simulink model "kapitsa"  (R2023b)
settings: Solver=VariableStepAuto  StartTime=0.0  StopTime=10.0  MaxStep=1e-4  RelTol=1e-3
undefined symbols (not defined in the file): f, I, l, m
settings Model: Creator=B03-304  LastModifiedBy=B03-304

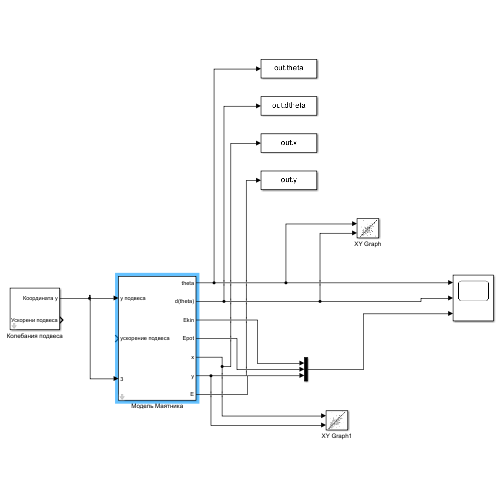
[thumbnail: Simulink's stored preview of the top-level diagram]
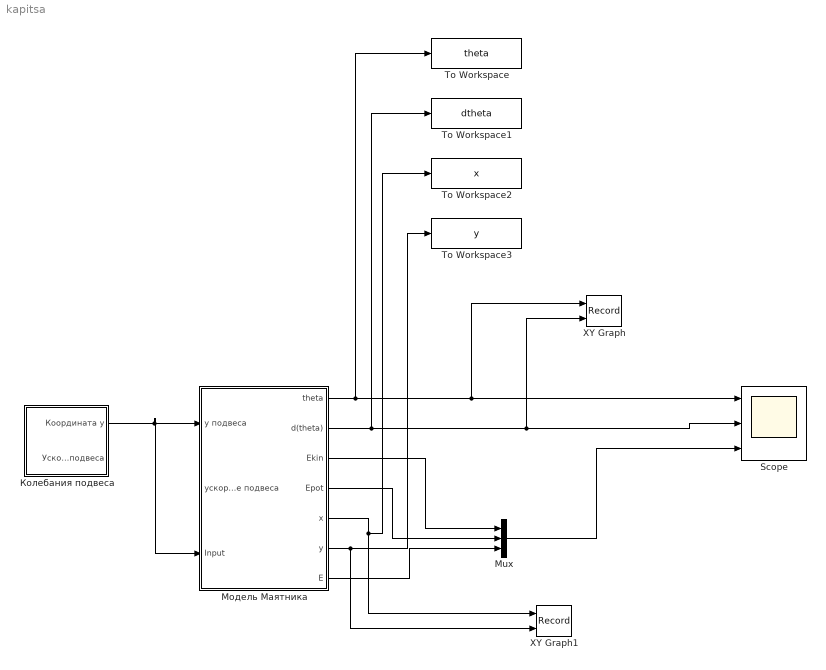
== system kapitsa ==
  Mux : Mux  Inputs=3
  Scope : Scope  NumInputPorts=3
  To Workspace : ToWorkspace  VariableName=theta  SampleTime=-1
  To Workspace1 : ToWorkspace  VariableName=dtheta  SampleTime=-1
  To Workspace2 : ToWorkspace  VariableName=x  SampleTime=-1
  To Workspace3 : ToWorkspace  VariableName=y  SampleTime=-1
  XY Graph : Record  FileSettingsInternal="{\"entries\":[{\"content\":{\"excelSettings\":{\"content\":{},\"type\":\"Streamout.ExcelSettings\"}},\"type\":\"Streamout.FileSettingStorage\",\"uuid\":\"\"}],\"packageUris\":[\"http:\\/\\/schema.mathworks.com\\/mf0\\/streamout_blocks\\/R2020a\"],\"version\":\"1.0\"}"  Layout=[1 1]  SignalsInternal="{\"entries\":[{\"content\":{\"signals\":[{\"content\":{\"blockPath\":[],\"dimensions\":[1],\"domain\":\"\",\"lineColor\":\"#a2142f\",\"plots\":[1],\"port\":1,\"sid\":[\"\"],\"signalID\":5426,\"signalName\":\"Модель Маятника:1\"},\"type\":\"RecordBlkView.Signal\",\"uuid\":\"\"},{\"content\":{\"blockPath\":[],\"dimensions\":[1],\"domain\":\"\",\"lineColor\":\"#139fff\",\"plots\":[1],\"port\":2,\"sid\":[\"\"],\"signalID\":5430,\"signalName\":\"Модель Маятника:2\"},\"type\":\"RecordBlkView.Signal\",\"uuid\":\"\"}]},\"type\":\"RecordBlkView.InputSignals\",\"uuid\":\"\"}],\"packageUris\":[\"http:\\/\\/schema.mathworks.com\\/mf0\\/streamout_blocks\\/R2020a\"],\"version\":\"1.0\"}"  VisualizationBindings="{\"xyplotplugin\":{\"info\":[{\"series\":[{\"bindingParametersList\":[{\"parameter\":\"X-Axis\",\"signalID\":5426,\"signalName\":\"Модель Маятника:1\"},{\"parameter\":\"Y-Axis\",\"signalID\":5430,\"signalName\":\"Модель Маятника:2\"}],\"seriesID\":46050}],\"subplotID\":1}]}}"  CompatibilityTag=XY
  XY Graph1 : Record  FileSettingsInternal="{\"entries\":[{\"content\":{\"excelSettings\":{\"content\":{},\"type\":\"Streamout.ExcelSettings\"}},\"type\":\"Streamout.FileSettingStorage\",\"uuid\":\"\"}],\"packageUris\":[\"http:\\/\\/schema.mathworks.com\\/mf0\\/streamout_blocks\\/R2020a\"],\"version\":\"1.0\"}"  Layout=[1 1]  SignalsInternal="{\"entries\":[{\"content\":{\"signals\":[{\"content\":{\"blockPath\":[],\"dimensions\":[1],\"domain\":\"\",\"lineColor\":\"#a2142f\",\"plots\":[1],\"port\":1,\"sid\":[\"\"],\"signalID\":5434,\"signalName\":\"Модель Маятника:5\"},\"type\":\"RecordBlkView.Signal\",\"uuid\":\"\"},{\"content\":{\"blockPath\":[],\"dimensions\":[1],\"domain\":\"\",\"lineColor\":\"#139fff\",\"plots\":[1],\"port\":2,\"sid\":[\"\"],\"signalID\":5438,\"signalName\":\"Модель Маятника:6\"},\"type\":\"RecordBlkView.Signal\",\"uuid\":\"\"}]},\"type\":\"RecordBlkView.InputSignals\",\"uuid\":\"\"}],\"packageUris\":[\"http:\\/\\/schema.mathworks.com\\/mf0\\/streamout_blocks\\/R2020a\"],\"version\":\"1.0\"}"  VisualizationBindings="{\"xyplotplugin\":{\"info\":[{\"series\":[{\"bindingParametersList\":[{\"parameter\":\"X-Axis\",\"signalID\":5434,\"signalName\":\"Модель Маятника:5\"},{\"parameter\":\"Y-Axis\",\"signalID\":5438,\"signalName\":\"Модель Маятника:6\"}],\"seriesID\":35113}],\"subplotID\":1}]}}"  CompatibilityTag=XY
  Колебания подвеса : Subsystem  mask{f=50, A=0.1}
  Модель Маятника : Subsystem  mask{thtea0=0, b=0, g=10}
  wires:
  Модель Маятника/1(theta) -> To Workspace/1, XY Graph/1, Scope/1
  Модель Маятника/2(d(theta)) -> XY Graph/2, Scope/2, To Workspace1/1
  Mux/1 -> Scope/3
  Модель Маятника/3(Ekin) -> Mux/1
  Модель Маятника/4(Epot) -> Mux/2
  Модель Маятника/7(E) -> Mux/3
  Модель Маятника/5(x) -> To Workspace2/1, XY Graph1/1
  Модель Маятника/6(y) -> XY Graph1/2, To Workspace3/1
  Колебания подвеса/1(Координата y) -> Модель Маятника/3(Input), Модель Маятника/1(y подвеса)

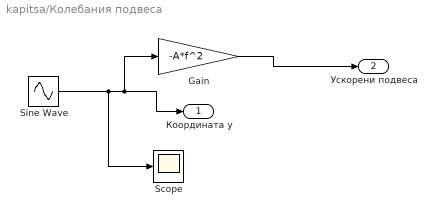
== system kapitsa/Колебания подвеса ==
  Gain : Gain  Gain=-A*f^2
  Scope : Scope
  Sine Wave : Sin  Amplitude=A  Frequency=f  Phase=pi/2  SampleTime=0
  Координата y : Outport
  Ускорени подвеса : Outport  Port=2
  wires:
  Sine Wave/1 -> Scope/1, Gain/1, Координата y/1
  Gain/1 -> Ускорени подвеса/1

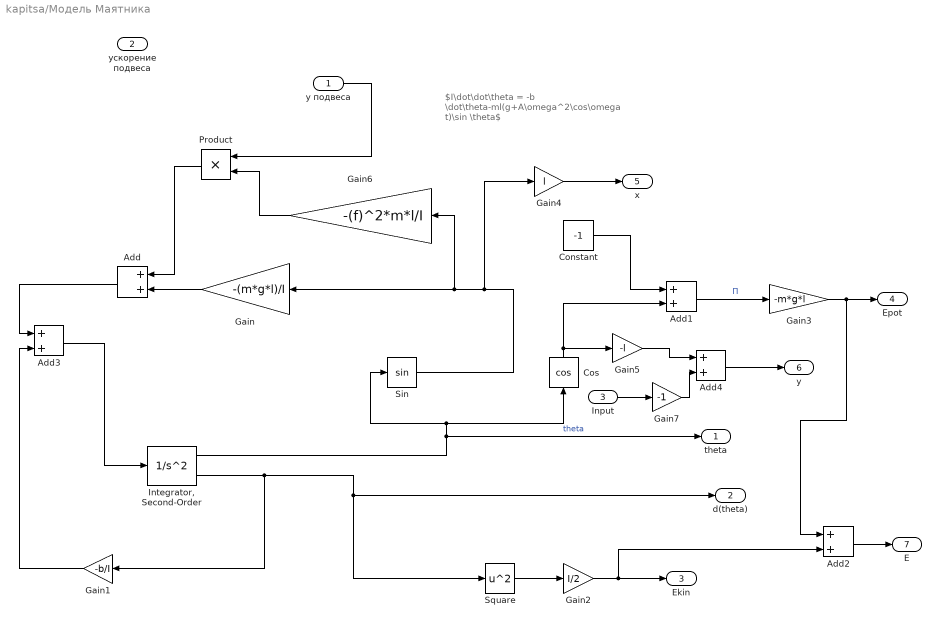
== system kapitsa/Модель Маятника ==
  note: $I\dot\dot\theta = -b \dot\theta-ml(g+A\omega^2\cos\omega t)\sin \theta$
  y подвеса : Inport
  ускорение подвеса : Inport  Port=2
  Input : Inport  Port=3
  Add{,1..4} (5 alike) : Sum
  Constant : Constant  Value=-1
  Cos : Trigonometry  Operator=cos
  Gain : Gain  Gain=-(m*g*l)/I
  Gain1 : Gain  Gain=-b/I
  Gain2 : Gain  Gain=I/2
  Gain3 : Gain  Gain=-m*g*l
  Gain4 : Gain  Gain=l
  Gain5 : Gain  Gain=-l
  Gain6 : Gain  Gain=-(f)^2*m*l/I
  Gain7 : Gain  Gain=-1
  "Integrator, Second-Order" : SecondOrderIntegrator  ICX=theta0  ICDXDT=0.1
  Product : Product
  Sin : Trigonometry
  Square : Math  Operator=square
  theta : Outport
  d(theta) : Outport  Port=2
  Ekin : Outport  Port=3
  Epot : Outport  Port=4
  x : Outport  Port=5
  y : Outport  Port=6
  E : Outport  Port=7
  wires:
  "Integrator, Second-Order"/1 -> theta/1, Cos/1, Sin/1  "theta"
  "Integrator, Second-Order"/2 -> Gain1/1, d(theta)/1, Square/1
  Square/1 -> Gain2/1
  Gain2/1 -> Add2/2, Ekin/1
  Cos/1 -> Gain5/1, Add1/2
  Constant/1 -> Add1/1
  Add1/1 -> Gain3/1  "П"
  Gain3/1 -> Add2/1, Epot/1
  Gain4/1 -> x/1
  Gain5/1 -> Add4/1
  Add2/1 -> E/1
  Gain1/1 -> Add3/2
  Add/1 -> Add3/1
  Gain/1 -> Add/2
  Sin/1 -> Gain4/1, Gain/1, Gain6/1
  Add3/1 -> "Integrator, Second-Order"/1
  y подвеса/1 -> Product/1
  Gain6/1 -> Product/2
  Product/1 -> Add/1
  Add4/1 -> y/1
  Input/1 -> Gain7/1
  Gain7/1 -> Add4/2
